simulink model "blob"  (R2019b)
settings: Solver=VariableStepAuto  StartTime=0.0  StopTime=10.0  RelTol=1e-3
libraries: visionsources x2
settings Model: Creator=Hritik Jaiswal  LastModifiedBy=Hritik Jaiswal

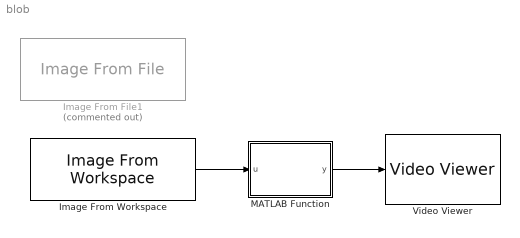
== system blob ==
  Image From File1 : visionsources/Image From File  Tag=vipblks_nd  Commented=on  FileName=F:\Opencv_Python\BlobsDemo.tif  Ts=inf  imagePorts=One multidimensional signal  OutPortLabels=R|G|B  ImageDataType=Inherit from input image  sdImageDataType=uint(8)  Signed=on  WordLength=16  FractionLengthMode=User-defined  FractionLength=15
      settings: SourceProductName=Computer Vision Toolbox
  Image From Workspace : visionsources/Image From Workspace  Tag=vipblks_nd  ImageValue=vidFrame1  Ts=inf  imagePorts=One multidimensional signal  OutPortLabels=R|G|B  ImageDataType=Inherit from 'Value'  Signed=on  WordLength=16  sdImageDataType=sfix(16)  FractionLengthMode=User-defined  FractionLength=15
      settings: SourceProductName=Computer Vision Toolbox  SourceProductBaseCode=VP
  MATLAB Function : MATLAB Function  TreatAsAtomicUnit=on
  Video Viewer : VideoViewer  FigPos=[1 766 1360 666]
  wires:
  Image From Workspace/1 -> MATLAB Function/1(u)
  MATLAB Function/1(y) -> Video Viewer/1

== matlab function blob/MATLAB Function ==
  data: u input; y output
function y = blob_detect(u)


%% Thresold image
I = rgb2hsv(u);

% Define thresholds for channel 1 based on histogram settings
channel1Min = 0.333;
channel1Max = 0.561;

% Define thresholds for channel 2 based on histogram settings
channel2Min = 0.327;
channel2Max = 1.000;

% Define thresholds for channel 3 based on histogram settings
channel3Min = 0.186;
channel3Max = 1.000;

% Create mask based on chosen histogram thresholds
sliderBW = (I(:,:,1) >= channel1Min ) & (I(:,:,1) <= channel1Max) & ...
    (I(:,:,2) >= channel2Min ) & (I(:,:,2) <= channel2Max) & ...
    (I(:,:,3) >= channel3Min ) & (I(:,:,3) <= channel3Max);
BW = sliderBW;


%% Remove disturbance
noise = strel('disk' , 3);

open = imopen(BW, noise);


%% blob analysis
blob = vision.BlobAnalysis('MinimumBlobArea',200,...    
    'MaximumBlobArea',5000);
% to perform a blob analysis on the video frame we need to use step
% function :- parameter => (blob analysis system object , input image i.e open)
% function output 3 :- area , centroid , bounding box

[~ , ~ , bboxout] = step(blob , open);

%% Anotate image

% now we get a bounding box cordinates of detected ball let apply contour
% over the detected ball using rectangle 

rectangle = insertShape(u , 'rectangle',bboxout , 'Linewidth' , 4 , 'Color',...
    [155 164 155]);


%% get the final result 


y = [u,rectangle];

end
